simulink model "MPC_Controller"  (Simulink 9.1)
settings: Solver=ode45  StartTime=0  StopTime=5  FixedStep=TSTEP  RelTol=1e-3  EnableMultiTasking=on
PreLoadFcn:
  | cd extensions\simulink\pt_center_diff
  | Run_ft4wd_eclass
  | lsd_parameta_eclass
  | cd ..\..\..
undefined symbols (not defined in the file): Theta, X, Y
libraries: robotlib x3, Solver_SF x1
settings Model: Creator=ywata  LastModifiedBy=xiaoyu  ExtModeTrigMode=oneshot  ExtModeArmWhenConnect=off
settings SolverCC: AlgebraicLoopSolver=LineSearch
settings DataIOCC: SignalLoggingSaveFormat=ModelDataLogs  SaveOutput=off  SaveTime=off  SignalLoggingName=sigsOut
settings OptimizationCC: BooleanDataType=off
settings DebuggingCC: SaveWithParameterizedLinksMsg=none  SignalResolutionControl=TryResolveAllWithWarning  MultiTaskDSMMsg=warning  MultiTaskCondExecSysMsg=none  FcnCallInpInsideContextMsg=warning  StateNameClashWarn=warning
settings HardwareCC: TargetBitPerPointer=64  TargetBitPerSizeT=64  TargetBitPerPtrDiffT=64  TargetLongLongMode=on  TargetIntDivRoundTo=Zero  TargetEndianess=LittleEndian  TargetWordSize=64  TargetHWDeviceType=MATLAB Host  ProdEqTarget=off
settings GRTTargetCC: TargetFcnLib=ansi_tfl_tmw.mat  ModelReferenceCompliant=off  MatFileLogging=off

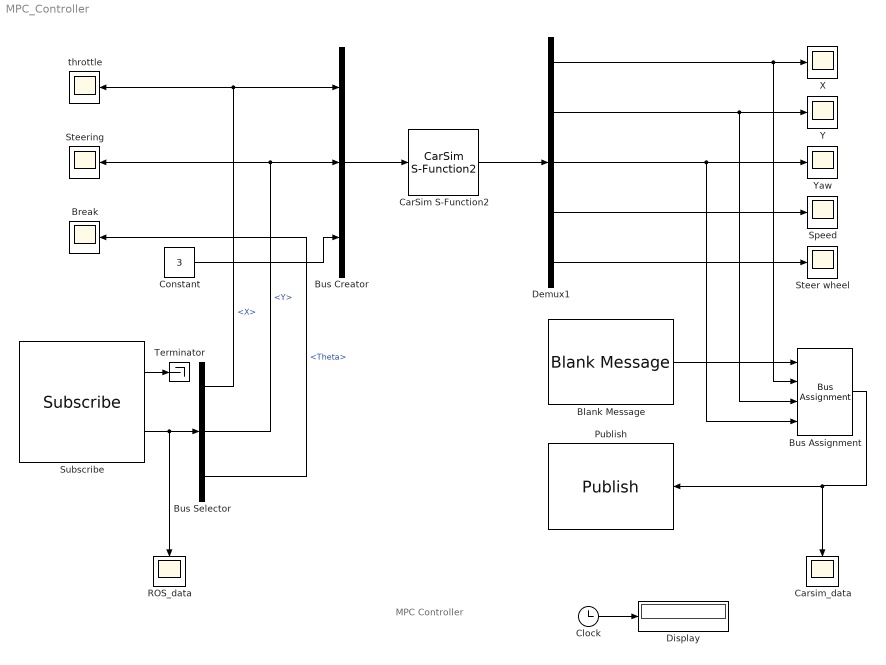
== system MPC_Controller ==
  note: MPC Controller
  Blank Message : robotlib/Blank Message  SourceLibraryInfo=This block requires Robotics System Toolbox  messageType=geometry_msgs/Pose2D  SampleTime=-1
      settings: SourceProductBaseCode=RO
  Break : Scope
  Bus Assignment : BusAssignment  AssignedSignals=X,Y,Theta
  Bus Creator : BusCreator  Inputs=3
  Bus Selector : BusSelector  OutputSignals=X,Y,Theta
  CarSim S-Function2 : Solver_SF/CarSim S-Function2  Priority=1  VehicleCode=i_s  SIMFILE=simfile.sim
      settings: AttributesFormatString=Vehicle Code: %<VehicleCode>
  Carsim_data : Scope
  Clock : Clock
  Constant : Constant  Value=3
  Demux1 : Demux  Outputs=5
  Display : Display
  Publish : robotlib/Publish  SourceLibraryInfo=This block requires Robotics System Toolbox  topicSource=Select from ROS network  topic=/simulink_pose  messageType=geometry_msgs/Pose2D  messageQueueLength=1
      settings: SourceProductBaseCode=RO
  ROS_data : Scope
  Speed : Scope
  Steer wheel : Scope
  Steering : Scope
  Subscribe : robotlib/Subscribe  SourceLibraryInfo=This block requires Robotics System Toolbox  topicSource=Select from ROS network  topic=/control  messageType=geometry_msgs/Pose2D  sampleTime=-1  messageQueueLength=3
      link override SourceBlock: ROSTopic=/control  ROSMessageType=std_msgs/Float64  SLBusName=SL_Bus_MPC_Controller_std_msgs_Float64  ModelName=MPC_Controller  BlockId=Sub_MPC_Controller_112
      settings: SourceProductBaseCode=RO
  Terminator : Terminator
  X : Scope
  Y : Scope
  Yaw : Scope
  throttle : Scope
  wires:
  Clock/1 -> Display/1
  Demux1/4 -> Speed/1
  Demux1/3 -> Bus Assignment/4, Yaw/1
  Demux1/2 -> Bus Assignment/3, Y/1
  Demux1/1 -> Bus Assignment/2, X/1
  Demux1/5 -> Steer wheel/1
  CarSim S-Function2/1 -> Demux1/1
  Bus Creator/1 -> CarSim S-Function2/1
  Subscribe/1 -> Terminator/1
  Subscribe/2 -> Bus Selector/1, ROS_data/1
  Blank Message/1 -> Bus Assignment/1
  Bus Assignment/1 -> Publish/1, Carsim_data/1
  Bus Selector/1 -> throttle/1, Bus Creator/1  "<X>"
  Bus Selector/2 -> Bus Creator/2, Steering/1  "<Y>"
  Bus Selector/3 -> Break/1  "<Theta>"
  Constant/1 -> Bus Creator/3
